simulink model "inverted_pendulum_controller"  (R2024a)
settings: Solver=VariableStepAuto  StartTime=0.0  StopTime=10  RelTol=1e-3
settings Model: Creator=amir  LastModifiedBy=amir

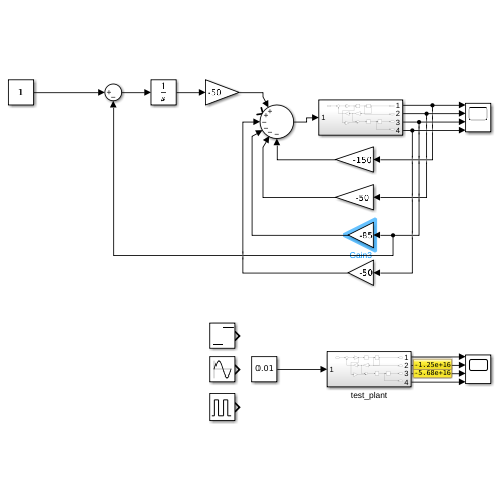
[thumbnail: Simulink's stored preview of the top-level diagram]
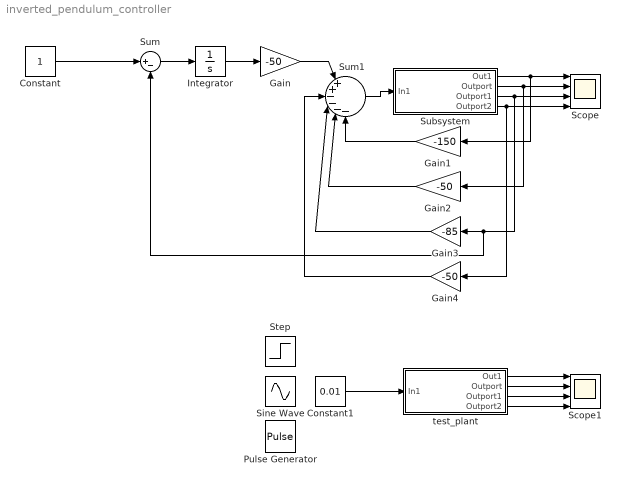
== system inverted_pendulum_controller ==
  Constant : Constant
  Constant1 : Constant  Value=0.01
  Gain : Gain  Gain=-50
  Gain1 : Gain  Gain=-150
  Gain2 : Gain  Gain=-50
  Gain3 : Gain  Gain=-85
  Gain4 : Gain  Gain=-50
  Integrator : Integrator
  Pulse Generator : DiscretePulseGenerator  PulseType=Time based  Amplitude=0.001  Period=1  PulseWidth=50
  Scope : Scope  NumInputPorts=4
  Scope1 : Scope  NumInputPorts=4
  Sine Wave : Sin  Amplitude=0.01  SampleTime=0
  Step : Step  Before=-0.01  After=0.01  SampleTime=0
  Subsystem : Subsystem
  Sum : Sum  Inputs=|+-
  Sum1 : Sum  Inputs=|++----
  test_plant : Subsystem
  wires:
  Subsystem/1(Out1) -> Gain1/1, Scope/1
  Subsystem/2(Outport) -> Gain2/1, Scope/2
  Subsystem/3(Outport1) -> Sum/2, Gain3/1, Scope/3
  Sum/1 -> Integrator/1
  Integrator/1 -> Gain/1
  Gain/1 -> Sum1/1
  Sum1/1 -> Subsystem/1(In1)
  Subsystem/4(Outport2) -> Gain4/1, Scope/4
  Gain1/1 -> Sum1/6
  Gain2/1 -> Sum1/5
  Gain3/1 -> Sum1/4
  Gain4/1 -> Sum1/3
  Constant/1 -> Sum/1
  test_plant/1(Out1) -> Scope1/1
  Constant1/1 -> test_plant/1(In1)
  test_plant/2(Outport) -> Scope1/2
  test_plant/3(Outport1) -> Scope1/3
  test_plant/4(Outport2) -> Scope1/4

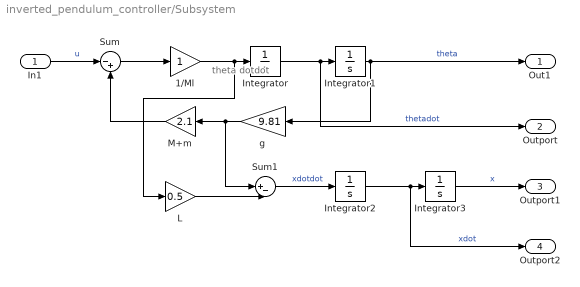
== system inverted_pendulum_controller/Subsystem ==
  note: theta
      | dotdot
  In1 : Inport
  1/Ml : Gain
  Integrator{,1..3} (4 alike) : Integrator
  L : Gain  Gain=0.5
  M+m : Gain  Gain=2.1
  Sum : Sum  Inputs=|-+
  Sum1 : Sum  Inputs=|+-
  g : Gain  Gain=9.81
  Out1 : Outport
  Outport : Outport  Port=2
  Outport1 : Outport  Port=3
  Outport2 : Outport  Port=4
  wires:
  In1/1 -> Sum/1  "u"
  Sum/1 -> 1/Ml/1
  1/Ml/1 -> L/1, Integrator/1
  Integrator/1 -> Outport/1, Integrator1/1  "thetadot"
  Integrator1/1 -> g/1, Out1/1  "theta"
  g/1 -> M+m/1, Sum1/1
  L/1 -> Sum1/2
  Integrator2/1 -> Outport2/1, Integrator3/1  "xdot"
  Sum1/1 -> Integrator2/1  "xdotdot"
  M+m/1 -> Sum/2
  Integrator3/1 -> Outport1/1  "x"

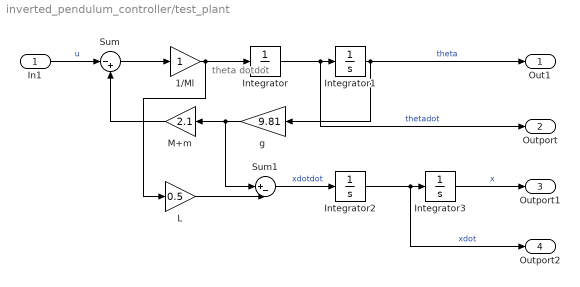
== system inverted_pendulum_controller/test_plant ==
  note: theta
      | dotdot
  In1 : Inport
  1/Ml : Gain
  Integrator{,1..3} (4 alike) : Integrator
  L : Gain  Gain=0.5
  M+m : Gain  Gain=2.1
  Sum : Sum  Inputs=|-+
  Sum1 : Sum  Inputs=|+-
  g : Gain  Gain=9.81
  Out1 : Outport
  Outport : Outport  Port=2
  Outport1 : Outport  Port=3
  Outport2 : Outport  Port=4
  wires:
  In1/1 -> Sum/1  "u"
  Sum/1 -> 1/Ml/1
  1/Ml/1 -> L/1, Integrator/1
  Integrator/1 -> Outport/1, Integrator1/1  "thetadot"
  Integrator1/1 -> g/1, Out1/1  "theta"
  g/1 -> M+m/1, Sum1/1
  L/1 -> Sum1/2
  Integrator3/1 -> Outport1/1  "x"
  Integrator2/1 -> Integrator3/1, Outport2/1  "xdot"
  Sum1/1 -> Integrator2/1  "xdotdot"
  M+m/1 -> Sum/2
